simulink model "CVCR"  (R2022a)
settings: Solver=VariableStepAuto  StartTime=0.0  StopTime=TsimTime  FixedStep=Tsim  MaxStep=Tsim*100  RelTol=1e-6
undefined symbols (not defined in the file): Cdc, Fpwm, Jt, Ke, Krpm, Kt, Ld, Ldc, Lq, P, Rdc, Re, RPM_slope, Tload, Tpwm, Tpwm_buck, Ts, Vdc_c
libraries: simulink x6
settings Model: Creator=MasterGnome  LastModifiedBy=MasterGnome
settings SolverCC: ZeroCrossAlgorithm=Adaptive
settings OptimizationCC: DefaultParameterBehavior=Inlined  EnhancedBackFolding=on  PassReuseOutputArgsAs=Individual arguments  ZeroExternalMemoryAtStartup=off  ZeroInternalMemoryAtStartup=off  OptimizeBlockOrder=speed  DifferentSizesBufferReuse=on  OptimizationCustomize=off  EfficientTunableParamExpr=on
settings DebuggingCC: IgnoredZcDiagnostic=none  ParameterTunabilityLossMsg=error  UnconnectedInputMsg=warning  UnconnectedOutputMsg=warning  UnconnectedLineMsg=warning
settings HardwareCC: ProdBitPerPointer=32  ProdBitPerSizeT=32  ProdBitPerPtrDiffT=32  ProdWordSize=32  ProdHWDeviceType=Intel->x86-32 (Windows32)  TargetBitPerPointer=64  TargetBitPerSizeT=64  TargetBitPerPtrDiffT=64  TargetLargestAtomicFloat=Float  TargetIntDivRoundTo=Zero  TargetEndianess=LittleEndian  TargetWordSize=64  TargetHWDeviceType=Intel->x86-64 (Windows64)
settings SFSimCC: MATLABDynamicMemAlloc=off
settings RTWCC: SystemTargetFile=ert.tlc  GenCodeOnly=on  TemplateMakefile=ert_default_tmf  DLArmComputeVersion=19.05
settings CodeAppCC: ForceParamTrailComments=on  IgnoreCustomStorageClasses=off  OperatorAnnotations=on  SimulinkDataObjDesc=on  SFDataObjDesc=on  InsertBlockDesc=on
settings ERTTargetCC: TargetLangStandard=C99 (ISO)  GenerateSampleERTMain=on  InlinedParameterPlacement=NonHierarchical  ERTCustomFileTemplate=example_file_process.tlc

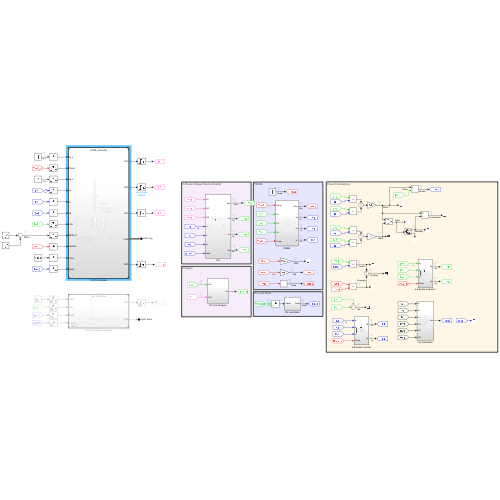
[thumbnail: Simulink's stored preview of the top-level diagram]
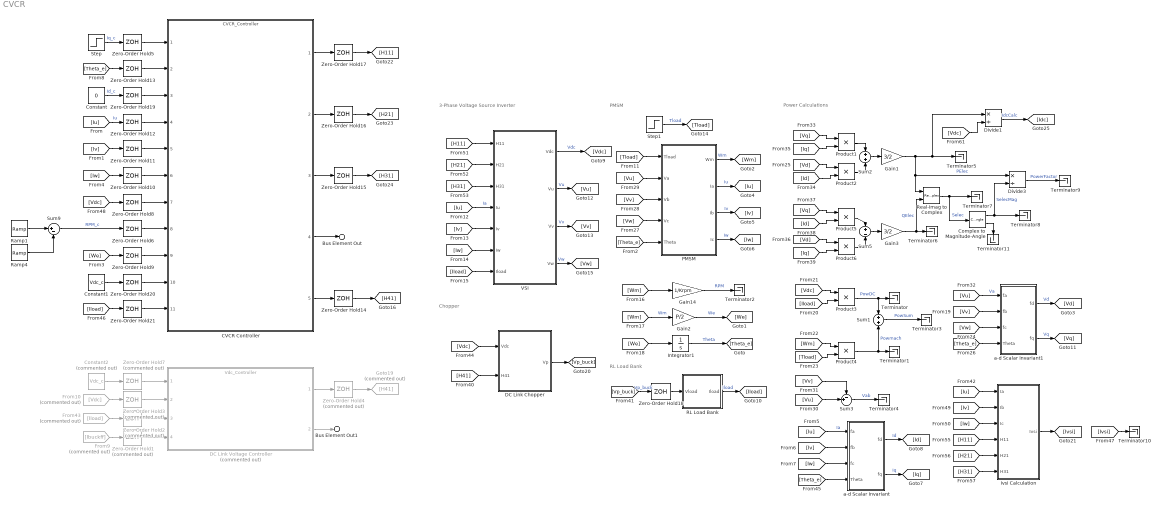
== system CVCR ==
  note: RL Load Bank
  note: Power Calculations
  note: PMSM
  note: 3-Phase Voltage Source Inverter
  note: Chopper
  CVCR Controller : ModelReference  ModelNameDialog=CVCR_Controller.slx  SimulationMode=Normal  ModelReferenceVersion=2.435
  Complex to Magnitude-Angle : ComplexToMagnitudeAngle
  Constant : Constant  Value=0
  Constant1 : Constant  Value=Vdc_c
  Constant2 : Constant  Commented=on  Value=Vdc_c
  DC Link Chopper : Subsystem
  DC Link Voltage Controller : ModelReference  Commented=on  ModelNameDialog=Vdc_Controller  SimulationMode=Normal  ModelReferenceVersion=2.345
  Divide1 : Product  Inputs=*/
  Divide3 : Product  Inputs=*/
  From10 : From  Commented=on  GotoTag=Vdc
  From43 : From  Commented=on  GotoTag=Iload
  From9 : From  Commented=on  GotoTag=Ibuckff
  Gain1 : Gain  Gain=3/2
  Gain14 : Gain  Gain=1/Krpm
  Gain2 : Gain  Gain=P/2
  Gain3 : Gain  Gain=3/2
  Goto19 : Goto  Commented=on  GotoTag=H41
  Integrator1 : Integrator
  Ivsi Calculation : Subsystem
  PMSM : Subsystem
  Product{1..6} (6 alike) : Product
  RL Load Bank : Subsystem
  Ramp1 : simulink/Sources/Ramp  slope=RPM_slope  start=RPM_Tstart  InitialOutput=0
  Ramp4 : simulink/Sources/Ramp  slope=RPM_slope  start=RPM_Tend  InitialOutput=0
  Real-Imag to Complex : RealImagToComplex
  Step : Step  Time=0.2  After=10  SampleTime=0
  Step1 : Step  Time=0.01  After=Tload  SampleTime=0
  Sum1 : Sum  Inputs=+|+
  Sum2 : Sum  Inputs=+|+
  Sum3 : Sum  Inputs=-+|
  Sum5 : Sum  Inputs=+|-
  Sum9 : Sum  Inputs=|+-
  Terminator{,1..11} (12 alike) : Terminator
  VSI : Subsystem
  Zero-Order Hold{1..4,7} (5 alike) : ZeroOrderHold  Commented=on  SampleTime=Ts
  Zero-Order Hold{5..6,8..21} (16 alike) : ZeroOrderHold  SampleTime=Ts
  a-d Scalar Invariant : Subsystem
  a-d Scalar Invariant1 : Subsystem
  Bus Element Out : Outport  PortName=LOG  Element=reg
  Bus Element Out1 : Outport  PortName=LOG  Element=buck
  wires:
  Gain14/1 -> Terminator2/1  "RPM"
  PMSM/1(Wm) -> [Wm]  "Wm"
  Step1/1 -> [Tload]  "Tload"
  Gain2/1 -> [We]  "We"
  PMSM/2(Ia) -> [Iu]  "Iu"
  PMSM/3(Ib) -> [Iv]  "Iv"
  PMSM/4(Ic) -> [Iw]  "Iw"
  Integrator1/1 -> [Theta_e]  "Theta"
  [Theta_e] -> PMSM/5(Theta)
  [Vdc] -> Product3/1
  [Iload] -> Product3/2
  Product3/1 -> Terminator/1, Sum1/1  "PowDC"
  Product4/1 -> Sum1/2, Terminator1/1  "Powmach"
  [Wm] -> Product4/1
  [Tload] -> Product4/2
  [Iv] -> VSI/5(Iv)
  [Iu] -> VSI/4(Iu)  "Ia"
  [Iw] -> VSI/6(Iw)
  VSI/1(Vdc) -> [Vdc]  "Vdc"
  [Tload] -> PMSM/1(Tload)
  [Wm] -> Gain14/1
  [Iload] -> VSI/7(Iload)
  From10/1 -> Zero-Order Hold3/1
  [Wm] -> Gain2/1  "Wm"
  [We] -> Integrator1/1
  Sum1/1 -> Terminator3/1  "PowSum"
  Sum3/1 -> Terminator4/1  "Vab"
  [Vv] -> a-d Scalar Invariant1/2(fb)
  [Theta_e] -> a-d Scalar Invariant1/4(Theta)
  a-d Scalar Invariant1/1(fd) -> [Vd]  "Vd"
  [Vw] -> a-d Scalar Invariant1/3(fc)
  a-d Scalar Invariant1/2(fq) -> [Vq]  "Vq"
  [Vu] -> a-d Scalar Invariant1/1(fa)  "Va"
  VSI/2(Vu) -> [Vu]  "Vu"
  VSI/3(Vv) -> [Vv]  "Vv"
  VSI/4(Vw) -> [Vw]  "Vw"
  [Vw] -> PMSM/4(Vc)
  [Vv] -> PMSM/3(Vb)
  [Vu] -> PMSM/2(Va)
  [Vu] -> Sum3/2
  [Vv] -> Sum3/1
  [Iq] -> Product1/2
  [Vq] -> Product1/1
  [Id] -> Product2/2
  [Vd] -> Product2/1
  Product1/1 -> Sum2/1
  Product2/1 -> Sum2/2
  Sum2/1 -> Gain1/1
  Product6/1 -> Sum5/2
  Product5/1 -> Sum5/1
  Gain3/1 -> Real-Imag to Complex/2, Terminator6/1  "QElec"
  [Vd] -> Product6/1
  [Vq] -> Product5/1
  Sum5/1 -> Gain3/1
  [Iq] -> Product6/2
  [Id] -> Product5/2
  Real-Imag to Complex/1 -> Complex to Magnitude-Angle/1, Terminator7/1  "Selec"
  Complex to Magnitude-Angle/1 -> Divide3/2, Terminator8/1  "SelecMag"
  Divide3/1 -> Terminator9/1  "PowerFactor"
  [H21] -> VSI/2(H21)
  [H31] -> VSI/3(H31)
  From43/1 -> Zero-Order Hold2/1
  RL Load Bank/1(Iload) -> [Iload]  "Iload"
  [H11] -> VSI/1(H11)
  Complex to Magnitude-Angle/2 -> Terminator11/1
  [Vp_buck] -> Zero-Order Hold18/1  "Vp_buck"
  DC Link Chopper/1(Vp) -> [Vp_buck]
  [Iu] -> Ivsi Calculation/1(Ia)
  [Iv] -> Ivsi Calculation/2(Ib)
  [Iw] -> Ivsi Calculation/3(Ic)
  [H11] -> Ivsi Calculation/4(H11)
  [H21] -> Ivsi Calculation/5(H21)
  [H31] -> Ivsi Calculation/6(H31)
  Ivsi Calculation/1(Ivsi) -> [Ivsi]
  From9/1 -> Zero-Order Hold1/1
  Divide1/1 -> [Idc]  "IdcCalc"
  Zero-Order Hold4/1 -> Goto19/1
  Gain1/1 -> Real-Imag to Complex/1, Divide3/1, Divide1/1, Terminator5/1  "PElec"
  [Vdc] -> Divide1/2
  Zero-Order Hold5/1 -> CVCR Controller/1
  [Theta_e] -> Zero-Order Hold13/1
  Constant/1 -> Zero-Order Hold19/1  "Id_c"
  [Iu] -> Zero-Order Hold12/1  "Iu"
  Constant2/1 -> Zero-Order Hold7/1
  Zero-Order Hold3/1 -> DC Link Voltage Controller/2
  Zero-Order Hold2/1 -> DC Link Voltage Controller/3
  Zero-Order Hold1/1 -> DC Link Voltage Controller/4
  DC Link Voltage Controller/1 -> Zero-Order Hold4/1
  CVCR Controller/3 -> Zero-Order Hold15/1
  CVCR Controller/2 -> Zero-Order Hold16/1
  CVCR Controller/1 -> Zero-Order Hold17/1
  a-d Scalar Invariant/1(fd) -> [Id]  "Id"
  a-d Scalar Invariant/2(fq) -> [Iq]  "Iq"
  [Iv] -> a-d Scalar Invariant/2(fb)
  [Iu] -> a-d Scalar Invariant/1(fa)  "Ia"
  [Iw] -> a-d Scalar Invariant/3(fc)
  [Theta_e] -> a-d Scalar Invariant/4(Theta)
  Zero-Order Hold15/1 -> [H31]
  Zero-Order Hold16/1 -> [H21]
  Zero-Order Hold17/1 -> [H11]
  Zero-Order Hold7/1 -> DC Link Voltage Controller/1
  [Ivsi] -> Terminator10/1
  Step/1 -> Zero-Order Hold5/1  "Iq_c"
  [Vdc] -> Zero-Order Hold8/1
  Zero-Order Hold13/1 -> CVCR Controller/2
  Zero-Order Hold19/1 -> CVCR Controller/3
  Zero-Order Hold12/1 -> CVCR Controller/4
  Zero-Order Hold11/1 -> CVCR Controller/5
  Zero-Order Hold10/1 -> CVCR Controller/6
  Zero-Order Hold8/1 -> CVCR Controller/7
  CVCR Controller/4 -> Bus Element Out/1
  [Iv] -> Zero-Order Hold11/1
  [Iw] -> Zero-Order Hold10/1
  Ramp1/1 -> Sum9/1
  Ramp4/1 -> Sum9/2
  Sum9/1 -> Zero-Order Hold6/1  "RPM_c"
  Zero-Order Hold6/1 -> CVCR Controller/8
  Zero-Order Hold9/1 -> CVCR Controller/9
  [We] -> Zero-Order Hold9/1
  Zero-Order Hold14/1 -> [H41]
  CVCR Controller/5 -> Zero-Order Hold14/1
  DC Link Voltage Controller/2 -> Bus Element Out1/1
  [Vdc] -> DC Link Chopper/1(Vdc)
  [H41] -> DC Link Chopper/2(H41)
  Zero-Order Hold18/1 -> RL Load Bank/1(Vload)
  Constant1/1 -> Zero-Order Hold20/1
  [Iload] -> Zero-Order Hold21/1
  Zero-Order Hold20/1 -> CVCR Controller/10
  Zero-Order Hold21/1 -> CVCR Controller/11

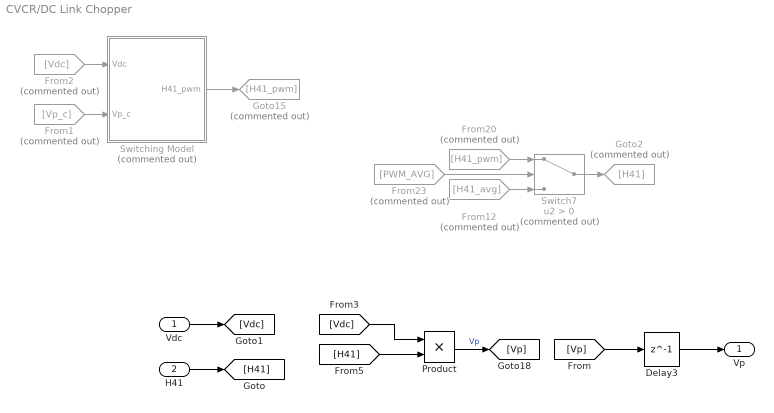
== system CVCR/DC Link Chopper ==
  Vdc : Inport
  H41 : Inport  Port=2
  Delay3 : Delay  DelayLength=1  InitialCondition=Vdc_c  SampleTime=Ts
  From1 : From  Commented=on  GotoTag=Vp_c
  From12 : From  Commented=on  GotoTag=H41_avg
  From2 : From  Commented=on  GotoTag=Vdc
  From20 : From  Commented=on  GotoTag=H41_pwm
  From23 : From  Commented=on  GotoTag=PWM_AVG
  Goto15 : Goto  Commented=on  GotoTag=H41_pwm
  Goto2 : Goto  Commented=on  GotoTag=H41
  Product : Product
  Switch7 : Switch  Commented=on  Criteria=u2 > Threshold  ZeroCross=off  SaturateOnIntegerOverflow=off  InputSameDT=off
  Switching Model : Subsystem  Commented=on
  Vp : Outport
  wires:
  H41/1 -> [H41]
  [Vp] -> Delay3/1
  Vdc/1 -> [Vdc]
  [Vdc] -> Product/1
  Product/1 -> [Vp]  "Vp"
  From20/1 -> Switch7/1
  From12/1 -> Switch7/3
  From23/1 -> Switch7/2
  Switching Model/1(H41_pwm) -> Goto15/1
  From2/1 -> Switching Model/1(Vdc)
  From1/1 -> Switching Model/2(Vp_c)
  Switch7/1 -> Goto2/1
  [H41] -> Product/2
  Delay3/1 -> Vp/1

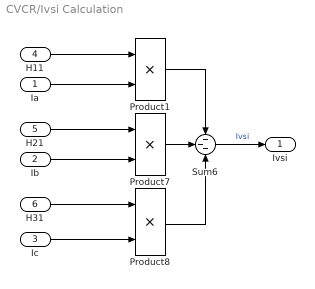
== system CVCR/Ivsi Calculation ==
  Ia : Inport
  Ib : Inport  Port=2
  Ic : Inport  Port=3
  H11 : Inport  Port=4
  H21 : Inport  Port=5
  H31 : Inport  Port=6
  Product1 : Product
  Product7 : Product
  Product8 : Product
  Sum6 : Sum  Inputs=---
  Ivsi : Outport
  wires:
  Ic/1 -> Product8/2
  Product8/1 -> Sum6/3
  H31/1 -> Product8/1
  Ib/1 -> Product7/2
  Product7/1 -> Sum6/2
  Product1/1 -> Sum6/1
  H11/1 -> Product1/1
  Sum6/1 -> Ivsi/1  "Ivsi"
  Ia/1 -> Product1/2
  H21/1 -> Product7/1

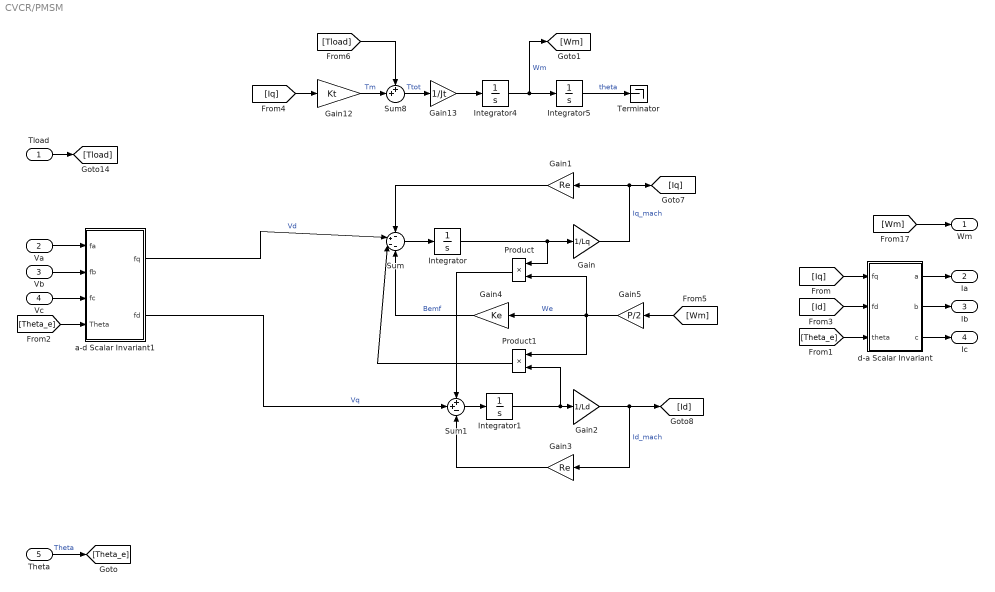
== system CVCR/PMSM ==
  Tload : Inport
  Va : Inport  Port=2
  Vb : Inport  Port=3
  Vc : Inport  Port=4
  Theta : Inport  Port=5
  Gain : Gain  Gain=1/Lq
  Gain1 : Gain  Gain=Re
  Gain12 : Gain  Gain=Kt
  Gain13 : Gain  Gain=1/Jt
  Gain2 : Gain  Gain=1/Ld
  Gain3 : Gain  Gain=Re
  Gain4 : Gain  Gain=Ke
  Gain5 : Gain  Gain=P/2
  Integrator : Integrator  InitialCondition=1
  Integrator1 : Integrator  InitialCondition=1
  Integrator4 : Integrator
  Integrator5 : Integrator
  Product : Product
  Product1 : Product
  Sum : Sum  Inputs=-+--
  Sum1 : Sum  Inputs=++-
  Sum8 : Sum  Inputs=++|
  Terminator : Terminator
  a-d Scalar Invariant1 : Subsystem
  d-a Scalar Invariant : Subsystem
  Wm : Outport
  Ia : Outport  Port=2
  Ib : Outport  Port=3
  Ic : Outport  Port=4
  wires:
  Sum1/1 -> Integrator1/1
  Gain5/1 -> Product1/1, Product/2, Gain4/1  "We"
  Gain1/1 -> Sum/1
  Integrator4/1 -> [Wm], Integrator5/1  "Wm"
  Sum8/1 -> Gain13/1  "Ttot"
  Integrator1/1 -> Product1/2, Gain2/1
  Gain3/1 -> Sum1/3
  [Tload] -> Sum8/1
  Integrator/1 -> Product/1, Gain/1
  Gain13/1 -> Integrator4/1
  Gain4/1 -> Sum/4  "Bemf"
  Sum/1 -> Integrator/1
  Product/1 -> Sum1/1
  Integrator5/1 -> Terminator/1  "theta"
  Product1/1 -> Sum/3
  d-a Scalar Invariant/3(c) -> Ic/1
  d-a Scalar Invariant/1(a) -> Ia/1
  Gain2/1 -> [Id], Gain3/1  "Id_mach"
  d-a Scalar Invariant/2(b) -> Ib/1
  Gain/1 -> [Iq], Gain1/1  "Iq_mach"
  Vc/1 -> a-d Scalar Invariant1/3(fc)
  Vb/1 -> a-d Scalar Invariant1/2(fb)
  Va/1 -> a-d Scalar Invariant1/1(fa)
  [Theta_e] -> a-d Scalar Invariant1/4(Theta)
  [Theta_e] -> d-a Scalar Invariant/3(theta)
  Theta/1 -> [Theta_e]  "Theta"
  [Iq] -> d-a Scalar Invariant/1(fq)
  [Id] -> d-a Scalar Invariant/2(fd)
  [Iq] -> Gain12/1
  Gain12/1 -> Sum8/2  "Tm"
  [Wm] -> Wm/1
  [Wm] -> Gain5/1
  Tload/1 -> [Tload]
  a-d Scalar Invariant1/1(fq) -> Sum/2  "Vd"
  a-d Scalar Invariant1/2(fd) -> Sum1/2  "Vq"

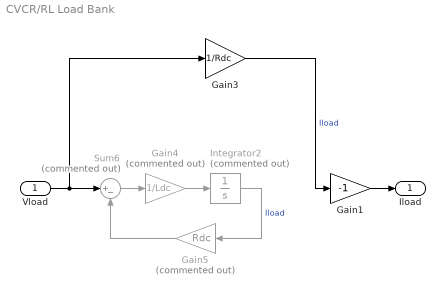
== system CVCR/RL Load Bank ==
  Vload : Inport
  Gain1 : Gain  Gain=-1
  Gain3 : Gain  Gain=1/Rdc
  Gain4 : Gain  Commented=on  Gain=1/Ldc
  Gain5 : Gain  Commented=on  Gain=Rdc
  Integrator2 : Integrator  Commented=on
  Sum6 : Sum  Commented=on  Inputs=|+-
  Iload : Outport
  wires:
  Gain5/1 -> Sum6/2
  Sum6/1 -> Gain4/1
  Vload/1 -> Gain3/1, Sum6/1
  Gain4/1 -> Integrator2/1
  Integrator2/1 -> Gain5/1  "Iload"
  Gain1/1 -> Iload/1
  Gain3/1 -> Gain1/1  "Iload"

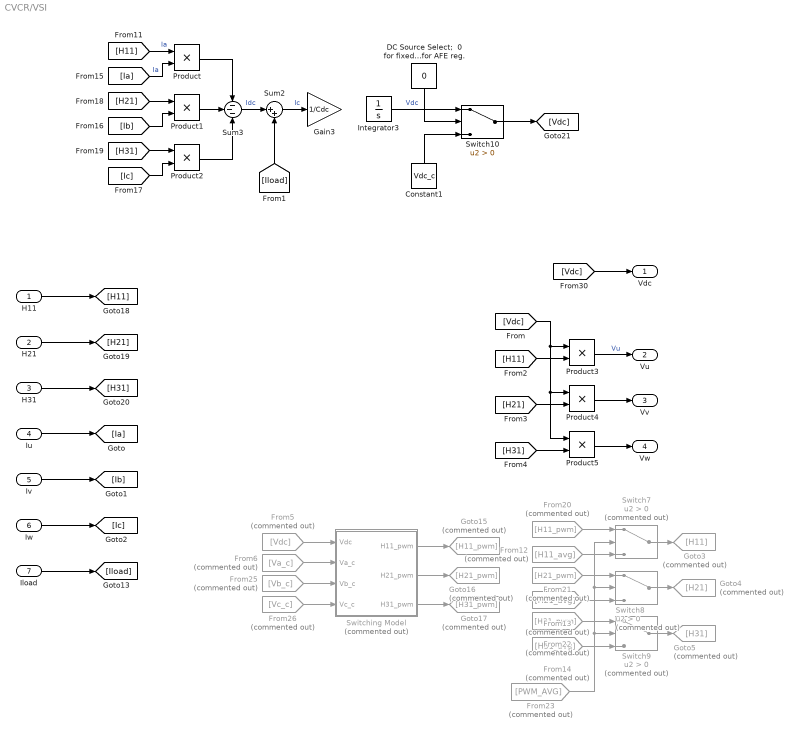
== system CVCR/VSI ==
  H11 : Inport
  H21 : Inport  Port=2
  H31 : Inport  Port=3
  Iu : Inport  Port=4
  Iv : Inport  Port=5
  Iw : Inport  Port=6
  Iload : Inport  Port=7
  Constant1 : Constant  Value=Vdc_c
  "DC Source Select;  0 for fixed, 1 for AFE reg." : Constant  Value=0
  From12 : From  Commented=on  GotoTag=H11_avg
  From13 : From  Commented=on  GotoTag=H21_avg
  From14 : From  Commented=on  GotoTag=H31_avg
  From20 : From  Commented=on  GotoTag=H11_pwm
  From21 : From  Commented=on  GotoTag=H21_pwm
  From22 : From  Commented=on  GotoTag=H31_pwm
  From23 : From  Commented=on  GotoTag=PWM_AVG
  From25 : From  Commented=on  GotoTag=Vb_c
  From26 : From  Commented=on  GotoTag=Vc_c
  From5 : From  Commented=on  GotoTag=Vdc
  From6 : From  Commented=on  GotoTag=Va_c
  Gain3 : Gain  Gain=1/Cdc
  Goto15 : Goto  Commented=on  GotoTag=H11_pwm
  Goto16 : Goto  Commented=on  GotoTag=H21_pwm
  Goto17 : Goto  Commented=on  GotoTag=H31_pwm
  Goto3 : Goto  Commented=on  GotoTag=H11
  Goto4 : Goto  Commented=on  GotoTag=H21
  Goto5 : Goto  Commented=on  GotoTag=H31
  Integrator3 : Integrator  InitialCondition=Vdc_c/3  UpperSaturationLimit=1500  LowerSaturationLimit=-1500
  Product{,1..5} (6 alike) : Product
  Sum2 : Sum  Inputs=|++
  Sum3 : Sum  Inputs=---
  Switch10 : Switch  Criteria=u2 > Threshold  ZeroCross=off  SaturateOnIntegerOverflow=off  InputSameDT=off
  Switch7 : Switch  Commented=on  Criteria=u2 > Threshold  ZeroCross=off  SaturateOnIntegerOverflow=off  InputSameDT=off
  Switch8 : Switch  Commented=on  Criteria=u2 > Threshold  ZeroCross=off  SaturateOnIntegerOverflow=off  InputSameDT=off
  Switch9 : Switch  Commented=on  Criteria=u2 > Threshold  ZeroCross=off  SaturateOnIntegerOverflow=off  InputSameDT=off
  Switching Model : Subsystem  Commented=on
  Vdc : Outport
  Vu : Outport  Port=2
  Vv : Outport  Port=3
  Vw : Outport  Port=4
  wires:
  Iload/1 -> [Iload]
  Sum3/1 -> Sum2/1  "Idc"
  H31/1 -> [H31]
  Sum2/1 -> Gain3/1  "Ic"
  H21/1 -> [H21]
  Product3/1 -> Vu/1  "Vu"
  [Ia] -> Product/2  "Ia"
  Product1/1 -> Sum3/2
  [Ib] -> Product1/2
  [H31] -> Product2/1
  [Ic] -> Product2/2
  Product2/1 -> Sum3/3
  [H21] -> Product1/1
  [Vdc] -> Vdc/1
  H11/1 -> [H11]
  [Vdc] -> Product3/1, Product5/1, Product4/1
  Product/1 -> Sum3/1
  [H11] -> Product/1  "Ia"
  Iv/1 -> [Ib]
  Iu/1 -> [Ia]
  Iw/1 -> [Ic]
  [Iload] -> Sum2/2
  Product4/1 -> Vv/1
  Product5/1 -> Vw/1
  Switch10/1 -> [Vdc]
  "DC Source Select;  0 for fixed, 1 for AFE reg."/1 -> Switch10/2
  Integrator3/1 -> Switch10/1  "Vdc"
  Constant1/1 -> Switch10/3
  [H11] -> Product3/2
  [H21] -> Product4/2
  [H31] -> Product5/2
  From26/1 -> Switching Model/4(Vc_c)
  From25/1 -> Switching Model/3(Vb_c)
  From5/1 -> Switching Model/1(Vdc)
  Switching Model/2(H21_pwm) -> Goto16/1
  Switching Model/1(H11_pwm) -> Goto15/1
  From6/1 -> Switching Model/2(Va_c)
  Switching Model/3(H31_pwm) -> Goto17/1
  From23/1 -> Switch7/2, Switch8/2, Switch9/2
  Switch9/1 -> Goto5/1
  From22/1 -> Switch9/1
  From21/1 -> Switch8/1
  Switch7/1 -> Goto3/1
  Switch8/1 -> Goto4/1
  From20/1 -> Switch7/1
  From12/1 -> Switch7/3
  From14/1 -> Switch9/3
  From13/1 -> Switch8/3

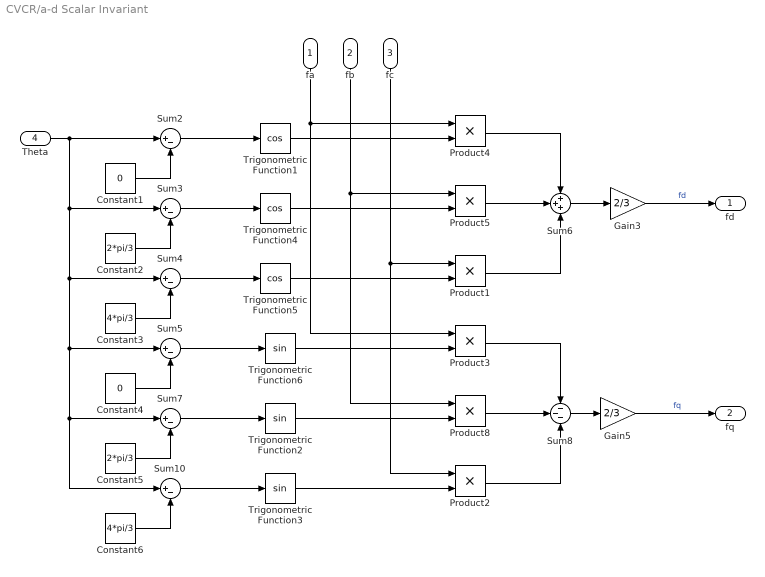
== system CVCR/a-d Scalar Invariant ==
  fa : Inport
  fb : Inport  Port=2
  fc : Inport  Port=3
  Theta : Inport  Port=4
  Constant1 : Constant  Value=0
  Constant2 : Constant  Value=2*pi/3
  Constant3 : Constant  Value=4*pi/3
  Constant4 : Constant  Value=0
  Constant5 : Constant  Value=2*pi/3
  Constant6 : Constant  Value=4*pi/3
  Gain3 : Gain  Gain=2/3
  Gain5 : Gain  Gain=2/3
  Product{1..5,8} (6 alike) : Product
  Sum{2..5,7,10} (6 alike) : Sum  Inputs=|+-
  Sum6 : Sum  Inputs=+++
  Sum8 : Sum  Inputs=---
  Trigonometric Function1 : Trigonometry  Operator=cos
  Trigonometric Function2 : Trigonometry
  Trigonometric Function3 : Trigonometry
  Trigonometric Function4 : Trigonometry  Operator=cos
  Trigonometric Function5 : Trigonometry  Operator=cos
  Trigonometric Function6 : Trigonometry
  fd : Outport
  fq : Outport  Port=2
  wires:
  Product1/1 -> Sum6/3
  fc/1 -> Product2/1, Product1/1
  Sum4/1 -> Trigonometric Function5/1
  Constant5/1 -> Sum7/2
  Trigonometric Function4/1 -> Product5/2
  Sum7/1 -> Trigonometric Function2/1
  Constant6/1 -> Sum10/2
  Trigonometric Function3/1 -> Product2/2
  Theta/1 -> Sum10/1, Sum7/1, Sum5/1, Sum4/1, Sum3/1, Sum2/1
  Sum10/1 -> Trigonometric Function3/1
  Sum5/1 -> Trigonometric Function6/1
  Product2/1 -> Sum8/3
  Trigonometric Function2/1 -> Product8/2
  Product3/1 -> Sum8/1
  Constant3/1 -> Sum4/2
  Trigonometric Function1/1 -> Product4/2
  Product8/1 -> Sum8/2
  Trigonometric Function5/1 -> Product1/2
  Constant2/1 -> Sum3/2
  Sum3/1 -> Trigonometric Function4/1
  Sum8/1 -> Gain5/1
  Constant4/1 -> Sum5/2
  Constant1/1 -> Sum2/2
  Sum2/1 -> Trigonometric Function1/1
  fa/1 -> Product4/1, Product3/1
  Gain3/1 -> fd/1  "fd"
  Sum6/1 -> Gain3/1
  Trigonometric Function6/1 -> Product3/2
  Product4/1 -> Sum6/1
  Gain5/1 -> fq/1  "fq"
  fb/1 -> Product5/1, Product8/1
  Product5/1 -> Sum6/2

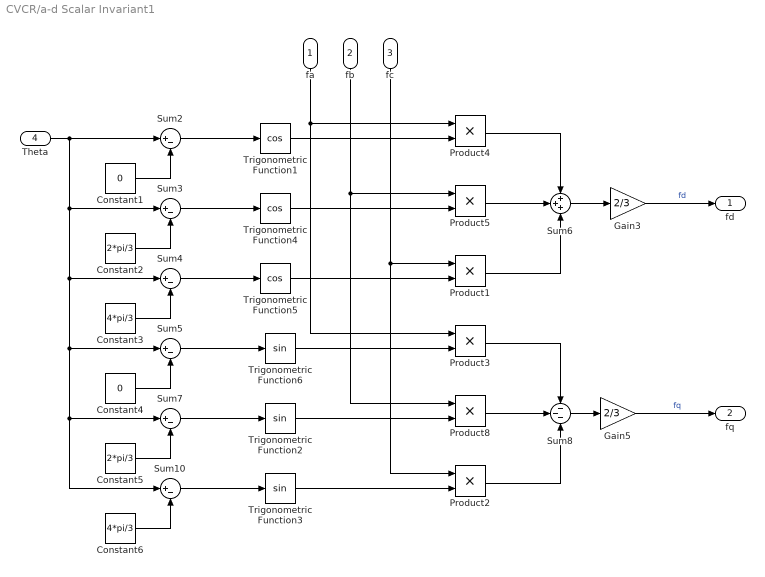
== system CVCR/a-d Scalar Invariant1 ==
  fa : Inport
  fb : Inport  Port=2
  fc : Inport  Port=3
  Theta : Inport  Port=4
  Constant1 : Constant  Value=0
  Constant2 : Constant  Value=2*pi/3
  Constant3 : Constant  Value=4*pi/3
  Constant4 : Constant  Value=0
  Constant5 : Constant  Value=2*pi/3
  Constant6 : Constant  Value=4*pi/3
  Gain3 : Gain  Gain=2/3
  Gain5 : Gain  Gain=2/3
  Product{1..5,8} (6 alike) : Product
  Sum{2..5,7,10} (6 alike) : Sum  Inputs=|+-
  Sum6 : Sum  Inputs=+++
  Sum8 : Sum  Inputs=---
  Trigonometric Function1 : Trigonometry  Operator=cos
  Trigonometric Function2 : Trigonometry
  Trigonometric Function3 : Trigonometry
  Trigonometric Function4 : Trigonometry  Operator=cos
  Trigonometric Function5 : Trigonometry  Operator=cos
  Trigonometric Function6 : Trigonometry
  fd : Outport
  fq : Outport  Port=2
  wires:
  Product1/1 -> Sum6/3
  fc/1 -> Product2/1, Product1/1
  Sum4/1 -> Trigonometric Function5/1
  Constant5/1 -> Sum7/2
  Trigonometric Function4/1 -> Product5/2
  Sum7/1 -> Trigonometric Function2/1
  Constant6/1 -> Sum10/2
  Trigonometric Function3/1 -> Product2/2
  Theta/1 -> Sum10/1, Sum7/1, Sum5/1, Sum4/1, Sum3/1, Sum2/1
  Sum10/1 -> Trigonometric Function3/1
  Sum5/1 -> Trigonometric Function6/1
  Product2/1 -> Sum8/3
  Trigonometric Function2/1 -> Product8/2
  Product3/1 -> Sum8/1
  Constant3/1 -> Sum4/2
  Trigonometric Function1/1 -> Product4/2
  Product8/1 -> Sum8/2
  Trigonometric Function5/1 -> Product1/2
  Constant2/1 -> Sum3/2
  Sum3/1 -> Trigonometric Function4/1
  Sum8/1 -> Gain5/1
  Constant4/1 -> Sum5/2
  Constant1/1 -> Sum2/2
  Sum2/1 -> Trigonometric Function1/1
  fa/1 -> Product4/1, Product3/1
  Gain3/1 -> fd/1  "fd"
  Sum6/1 -> Gain3/1
  Trigonometric Function6/1 -> Product3/2
  Product4/1 -> Sum6/1
  Gain5/1 -> fq/1  "fq"
  fb/1 -> Product5/1, Product8/1
  Product5/1 -> Sum6/2

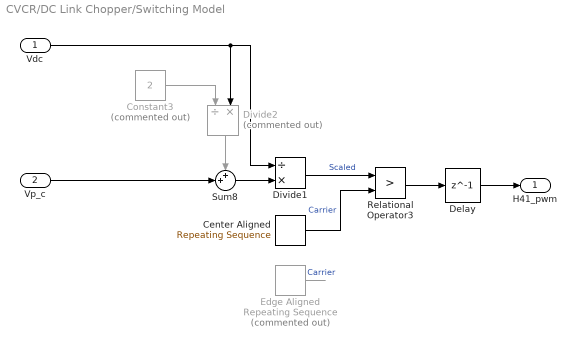
== system CVCR/DC Link Chopper/Switching Model ==
  Vdc : Inport
  Vp_c : Inport  Port=2
  Center Aligned : simulink/Sources/Repeating Sequence  rep_seq_t=[0 1/(2*Fpwm) 1/Fpwm]  rep_seq_y=[0 1 0]
  Constant3 : Constant  Commented=on  Value=2
  Delay : Delay  DelayLength=1  SampleTime=Tpwm_buck
  Divide1 : Product  Inputs=/*
  Divide2 : Product  Commented=on  Inputs=/*
  Edge Aligned : simulink/Sources/Repeating Sequence  Commented=on  rep_seq_t=[0 1/Fpwm]  rep_seq_y=[0 1]
  Relational Operator3 : RelationalOperator  Operator=>  OutDataTypeStr=boolean  ZeroCross=off  RndMeth=Simplest  InputSameDT=off
  Sum8 : Sum  Inputs=++|
  H41_pwm : Outport
  wires:
  Divide1/1 -> Relational Operator3/1  "Scaled"
  Center Aligned/1 -> Relational Operator3/2  "Carrier"
  Divide2/1 -> Sum8/1
  Vdc/1 -> Divide1/1, Divide2/2
  Edge Aligned/1 -> ?  "Carrier"
  Constant3/1 -> Divide2/1
  Sum8/1 -> Divide1/2
  Vp_c/1 -> Sum8/2
  Relational Operator3/1 -> Delay/1
  Delay/1 -> H41_pwm/1

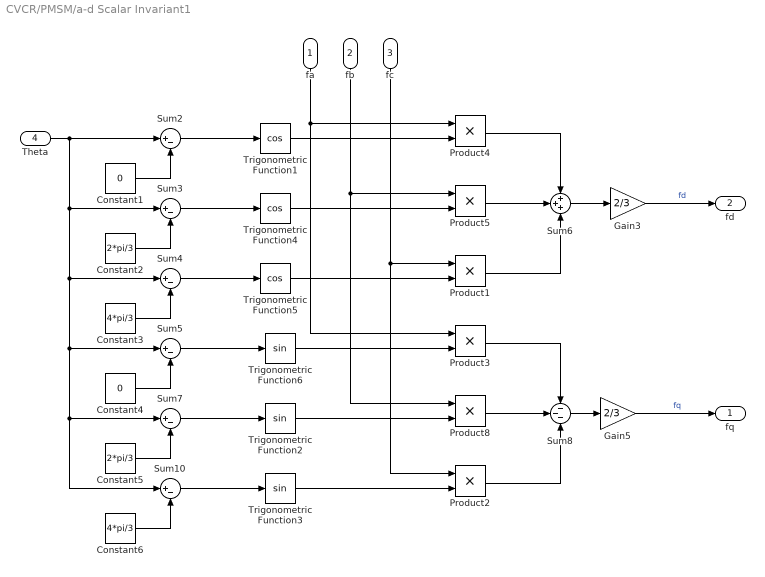
== system CVCR/PMSM/a-d Scalar Invariant1 ==
  fa : Inport
  fb : Inport  Port=2
  fc : Inport  Port=3
  Theta : Inport  Port=4
  Constant1 : Constant  Value=0
  Constant2 : Constant  Value=2*pi/3
  Constant3 : Constant  Value=4*pi/3
  Constant4 : Constant  Value=0
  Constant5 : Constant  Value=2*pi/3
  Constant6 : Constant  Value=4*pi/3
  Gain3 : Gain  Gain=2/3
  Gain5 : Gain  Gain=2/3
  Product{1..5,8} (6 alike) : Product
  Sum{2..5,7,10} (6 alike) : Sum  Inputs=|+-
  Sum6 : Sum  Inputs=+++
  Sum8 : Sum  Inputs=---
  Trigonometric Function1 : Trigonometry  Operator=cos
  Trigonometric Function2 : Trigonometry
  Trigonometric Function3 : Trigonometry
  Trigonometric Function4 : Trigonometry  Operator=cos
  Trigonometric Function5 : Trigonometry  Operator=cos
  Trigonometric Function6 : Trigonometry
  fq : Outport
  fd : Outport  Port=2
  wires:
  Product1/1 -> Sum6/3
  fc/1 -> Product2/1, Product1/1
  Sum4/1 -> Trigonometric Function5/1
  Constant5/1 -> Sum7/2
  Trigonometric Function4/1 -> Product5/2
  Sum7/1 -> Trigonometric Function2/1
  Constant6/1 -> Sum10/2
  Trigonometric Function3/1 -> Product2/2
  Theta/1 -> Sum10/1, Sum7/1, Sum5/1, Sum4/1, Sum3/1, Sum2/1
  Sum10/1 -> Trigonometric Function3/1
  Sum5/1 -> Trigonometric Function6/1
  Product2/1 -> Sum8/3
  Trigonometric Function2/1 -> Product8/2
  Product3/1 -> Sum8/1
  Constant3/1 -> Sum4/2
  Trigonometric Function1/1 -> Product4/2
  Product8/1 -> Sum8/2
  Trigonometric Function5/1 -> Product1/2
  Constant2/1 -> Sum3/2
  Sum3/1 -> Trigonometric Function4/1
  Sum8/1 -> Gain5/1
  Constant4/1 -> Sum5/2
  Constant1/1 -> Sum2/2
  Sum2/1 -> Trigonometric Function1/1
  fa/1 -> Product4/1, Product3/1
  Gain3/1 -> fd/1  "fd"
  Sum6/1 -> Gain3/1
  Trigonometric Function6/1 -> Product3/2
  Product4/1 -> Sum6/1
  Gain5/1 -> fq/1  "fq"
  fb/1 -> Product5/1, Product8/1
  Product5/1 -> Sum6/2

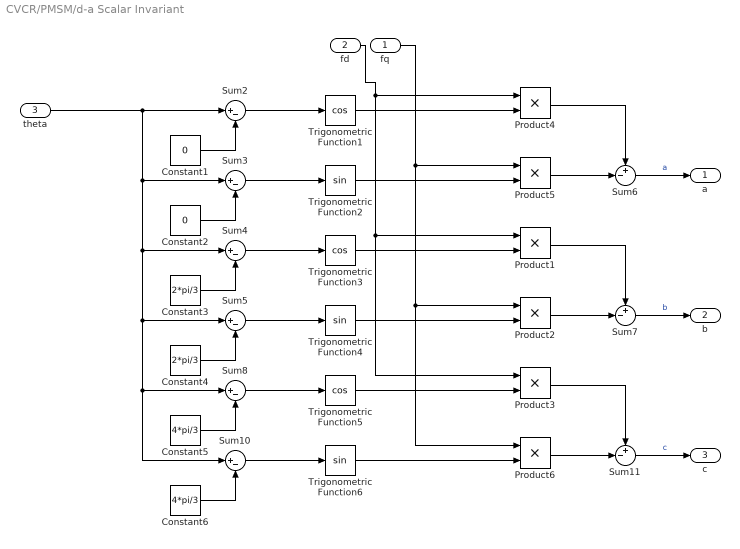
== system CVCR/PMSM/d-a Scalar Invariant ==
  fq : Inport
  fd : Inport  Port=2
  theta : Inport  Port=3
  Constant1 : Constant  Value=0
  Constant2 : Constant  Value=0
  Constant3 : Constant  Value=2*pi/3
  Constant4 : Constant  Value=2*pi/3
  Constant5 : Constant  Value=4*pi/3
  Constant6 : Constant  Value=4*pi/3
  Product{1..6} (6 alike) : Product
  Sum{2..5,8,10} (6 alike) : Sum  Inputs=|+-
  Sum11 : Sum  Inputs=+-|
  Sum6 : Sum  Inputs=+-|
  Sum7 : Sum  Inputs=+-|
  Trigonometric Function1 : Trigonometry  Operator=cos
  Trigonometric Function2 : Trigonometry
  Trigonometric Function3 : Trigonometry  Operator=cos
  Trigonometric Function4 : Trigonometry
  Trigonometric Function5 : Trigonometry  Operator=cos
  Trigonometric Function6 : Trigonometry
  a : Outport
  b : Outport  Port=2
  c : Outport  Port=3
  wires:
  theta/1 -> Sum2/1, Sum3/1, Sum4/1, Sum5/1, Sum8/1, Sum10/1
  Trigonometric Function6/1 -> Product6/2
  Trigonometric Function5/1 -> Product3/2
  Constant4/1 -> Sum5/2
  Product1/1 -> Sum7/1
  Trigonometric Function1/1 -> Product4/2
  Product6/1 -> Sum11/2
  Sum10/1 -> Trigonometric Function6/1
  fd/1 -> Product3/1, Product1/1, Product4/1
  Sum3/1 -> Trigonometric Function2/1
  fq/1 -> Product6/1, Product2/1, Product5/1
  Product5/1 -> Sum6/2
  Trigonometric Function2/1 -> Product5/2
  Constant6/1 -> Sum10/2
  Sum8/1 -> Trigonometric Function5/1
  Sum2/1 -> Trigonometric Function1/1
  Sum4/1 -> Trigonometric Function3/1
  Constant1/1 -> Sum2/2
  Product2/1 -> Sum7/2
  Trigonometric Function3/1 -> Product1/2
  Sum5/1 -> Trigonometric Function4/1
  Trigonometric Function4/1 -> Product2/2
  Constant5/1 -> Sum8/2
  Sum6/1 -> a/1  "a"
  Constant3/1 -> Sum4/2
  Product3/1 -> Sum11/1
  Product4/1 -> Sum6/1
  Constant2/1 -> Sum3/2
  Sum11/1 -> c/1  "c"
  Sum7/1 -> b/1  "b"

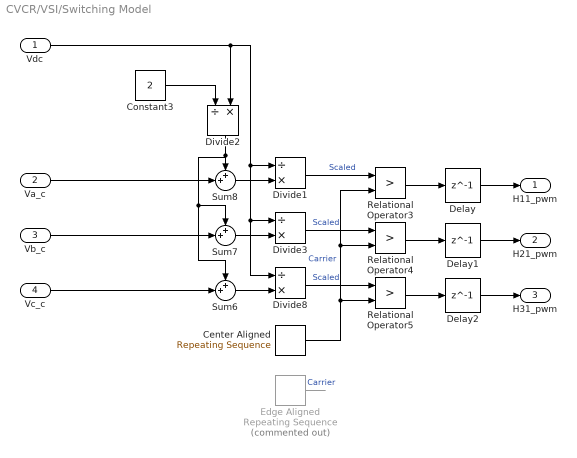
== system CVCR/VSI/Switching Model ==
  Vdc : Inport
  Va_c : Inport  Port=2
  Vb_c : Inport  Port=3
  Vc_c : Inport  Port=4
  Center Aligned : simulink/Sources/Repeating Sequence  rep_seq_t=[0 1/(2*Fpwm) 1/Fpwm]  rep_seq_y=[0 1 0]
  Constant3 : Constant  Value=2
  Delay : Delay  DelayLength=1  SampleTime=Tpwm
  Delay1 : Delay  DelayLength=1  SampleTime=Tpwm
  Delay2 : Delay  DelayLength=1  SampleTime=Tpwm
  Divide{1..3,8} (4 alike) : Product  Inputs=/*
  Edge Aligned : simulink/Sources/Repeating Sequence  Commented=on  rep_seq_t=[0 1/Fpwm]  rep_seq_y=[0 1]
  Relational Operator3 : RelationalOperator  Operator=>  OutDataTypeStr=boolean  ZeroCross=off  RndMeth=Simplest  InputSameDT=off
  Relational Operator4 : RelationalOperator  Operator=>  OutDataTypeStr=boolean  ZeroCross=off  RndMeth=Simplest  InputSameDT=off
  Relational Operator5 : RelationalOperator  Operator=>  OutDataTypeStr=boolean  ZeroCross=off  RndMeth=Simplest  InputSameDT=off
  Sum6 : Sum  Inputs=++|
  Sum7 : Sum  Inputs=++|
  Sum8 : Sum  Inputs=++|
  H11_pwm : Outport
  H21_pwm : Outport  Port=2
  H31_pwm : Outport  Port=3
  wires:
  Delay1/1 -> H21_pwm/1
  Delay/1 -> H11_pwm/1
  Delay2/1 -> H31_pwm/1
  Relational Operator5/1 -> Delay2/1
  Relational Operator3/1 -> Delay/1
  Vb_c/1 -> Sum7/2
  Va_c/1 -> Sum8/2
  Vc_c/1 -> Sum6/2
  Sum8/1 -> Divide1/2
  Divide3/1 -> Relational Operator4/1  "Scaled"
  Sum6/1 -> Divide8/2
  Divide8/1 -> Relational Operator5/1  "Scaled"
  Constant3/1 -> Divide2/1
  Sum7/1 -> Divide3/2
  Edge Aligned/1 -> ?  "Carrier"
  Relational Operator4/1 -> Delay1/1
  Vdc/1 -> Divide2/2, Divide1/1, Divide3/1, Divide8/1
  Divide2/1 -> Sum8/1, Sum7/1, Sum6/1
  Center Aligned/1 -> Relational Operator5/2, Relational Operator4/2, Relational Operator3/2  "Carrier"
  Divide1/1 -> Relational Operator3/1  "Scaled"
